simulink model "Obstacle_Detection"  (R2017b)
settings: configuration reference "Autosar_CodeGeneration" (kept outside this file)
settings Model: RequirementInfo={'linktype_rmi_url' 'http://md1hxhhc.ww004.siemens.net/polarion/' '@/project/ATRover/workitem?id=ATR-528' 'true' 'Polarion: ATR-528' '' } %GIDa_54e2749a_9850_4405_b077_57153701a047  DataDictionary=RoverDataDict.sldd  Creator=sam  LastModifiedBy=eh6qym
settings ConfigSetRef: DDName=RoverDataDict.sldd

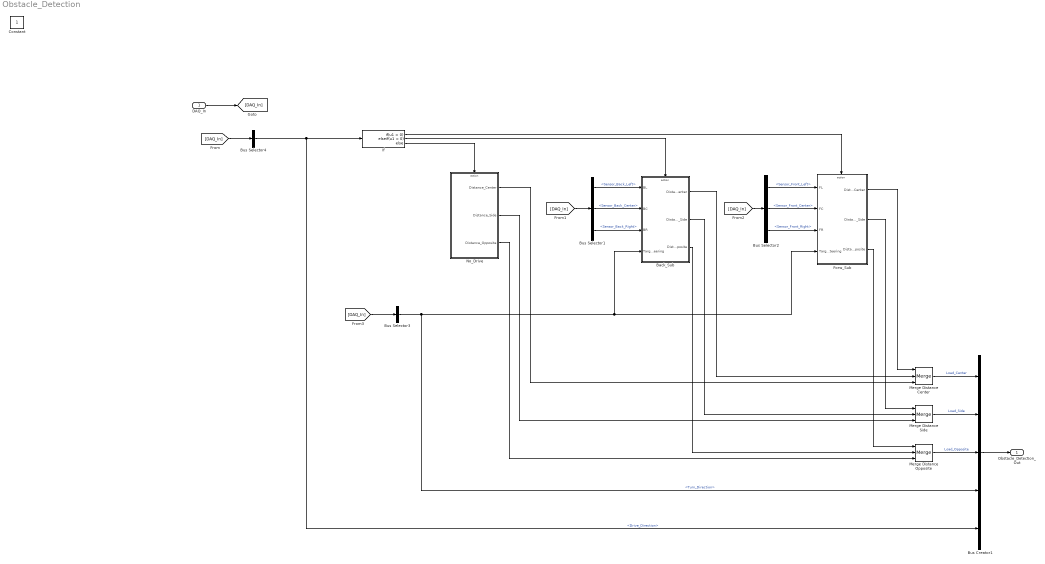
== system Obstacle_Detection ==
  DAQ_In : Inport  OutDataTypeStr=Bus: DAQ_In
  Back_Sub : Subsystem  TreatAsAtomicUnit=on
  Bus Creator1 : BusCreator  Inputs=5  OutDataTypeStr=Bus: Obstacle_Detection_Out  NonVirtualBus=on
      settings: InheritFromInputs=off
  Bus Selector1 : BusSelector  OutputSignals=Sensor_Back_Left,Sensor_Back_Center,Sensor_Back_Right
  Bus Selector2 : BusSelector  OutputSignals=Sensor_Front_Left,Sensor_Front_Center,Sensor_Front_Right
  Bus Selector3 : BusSelector  OutputSignals=Turn_Direction
  Bus Selector4 : BusSelector  OutputSignals=Drive_Direction
  Forw_Sub : Subsystem  TreatAsAtomicUnit=on
  If : If  ElseIfExpressions=u1 < 0
  Merge Distance Center : Merge  Inputs=3
  Merge Distance Opposite : Merge  Inputs=3
  Merge Distance Side : Merge  Inputs=3
  No_Drive : Subsystem  TreatAsAtomicUnit=on
  Obstacle_Detection_Out : Outport  OutDataTypeStr=Bus: Obstacle_Detection_Out
  Constant : Constant  IOType=siggen
  wires:
  Bus Creator1/1 -> Obstacle_Detection_Out/1
  Bus Selector1/1 -> Back_Sub/1(BL)  "<Sensor_Back_Left>"
  Bus Selector1/2 -> Back_Sub/2(BC)  "<Sensor_Back_Center>"
  Bus Selector1/3 -> Back_Sub/3(BR)  "<Sensor_Back_Right>"
  Bus Selector2/1 -> Forw_Sub/1(FL)  "<Sensor_Front_Left>"
  Bus Selector2/2 -> Forw_Sub/2(FC)  "<Sensor_Front_Center>"
  Bus Selector2/3 -> Forw_Sub/3(FR)  "<Sensor_Front_Right>"
  Bus Selector3/1 -> Bus Creator1/4, Forw_Sub/4(Target_Steering), Back_Sub/4(Target_Steering)  "<Turn_Direction>"
  Forw_Sub/2(Distance_Side) -> Merge Distance Side/1
  Back_Sub/2(Distance_Side) -> Merge Distance Side/2
  Merge Distance Side/1 -> Bus Creator1/2  "Load_Side"
  DAQ_In/1 -> [DAQ_In]
  [DAQ_In] -> Bus Selector4/1
  [DAQ_In] -> Bus Selector1/1
  [DAQ_In] -> Bus Selector2/1
  [DAQ_In] -> Bus Selector3/1
  Merge Distance Center/1 -> Bus Creator1/1  "Load_Center"
  Back_Sub/1(Distance_Center) -> Merge Distance Center/2
  Forw_Sub/1(Distance_Center) -> Merge Distance Center/1
  Bus Selector4/1 -> Bus Creator1/5, If/1  "<Drive_Direction>"
  If/1 -> Forw_Sub/Action
  If/2 -> Back_Sub/Action
  Merge Distance Opposite/1 -> Bus Creator1/3  "Load_Opposite"
  Forw_Sub/3(Distance_Opposite) -> Merge Distance Opposite/1
  Back_Sub/3(Distance_Opposite) -> Merge Distance Opposite/2
  If/3 -> No_Drive/Action
  No_Drive/1(Distance_Center) -> Merge Distance Center/3
  No_Drive/2(Distance_Side) -> Merge Distance Side/3
  No_Drive/3(Distance_Opposite) -> Merge Distance Opposite/3

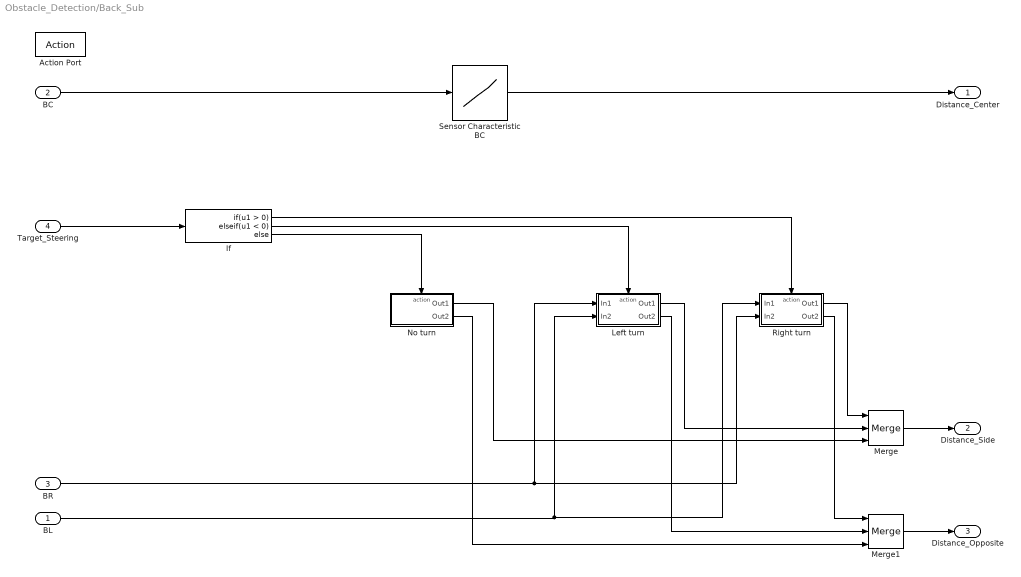
== system Obstacle_Detection/Back_Sub ==
  BL : Inport  OutDataTypeStr=double
  BC : Inport  Port=2  OutDataTypeStr=double
  BR : Inport  Port=3  OutDataTypeStr=double
  Target_Steering : Inport  Port=4  OutDataTypeStr=double
  Action Port : ActionPort  ActionType=elseif
  If : If  ElseIfExpressions=u1 < 0
  Left turn : Subsystem  TreatAsAtomicUnit=on
  Merge : Merge  Inputs=3
  Merge1 : Merge  Inputs=3
  No turn : Subsystem  TreatAsAtomicUnit=on
  Right turn : Subsystem  TreatAsAtomicUnit=on
  Sensor Characteristic BC : Lookup_n-D  NumberOfTableDimensions=1  BreakpointsForDimension1=[0.06 0.15 0.26 0.6 0.64]  Table=[0.80 0.40 0.20 0.07 0.06]  RemoveProtectionInput=on  InternalRulePriority=Speed  RndMeth=Simplest  InputSameDT=on
  Distance_Center : Outport  InitialOutput=[0.8]
  Distance_Side : Outport  Port=2  OutDataTypeStr=double  InitialOutput=[0.8]
  Distance_Opposite : Outport  Port=3  OutDataTypeStr=double  InitialOutput=[0.8]
  wires:
  BC/1 -> Sensor Characteristic BC/1
  Sensor Characteristic BC/1 -> Distance_Center/1
  Merge/1 -> Distance_Side/1
  BR/1 -> Right turn/2(In2), Left turn/1(In1)
  BL/1 -> Left turn/2(In2), Right turn/1(In1)
  Left turn/1(Out1) -> Merge/2
  Right turn/1(Out1) -> Merge/1
  If/1 -> Right turn/Action
  If/2 -> Left turn/Action
  Merge1/1 -> Distance_Opposite/1
  Left turn/2(Out2) -> Merge1/2
  Right turn/2(Out2) -> Merge1/1
  If/3 -> No turn/Action
  No turn/1(Out1) -> Merge/3
  No turn/2(Out2) -> Merge1/3
  Target_Steering/1 -> If/1

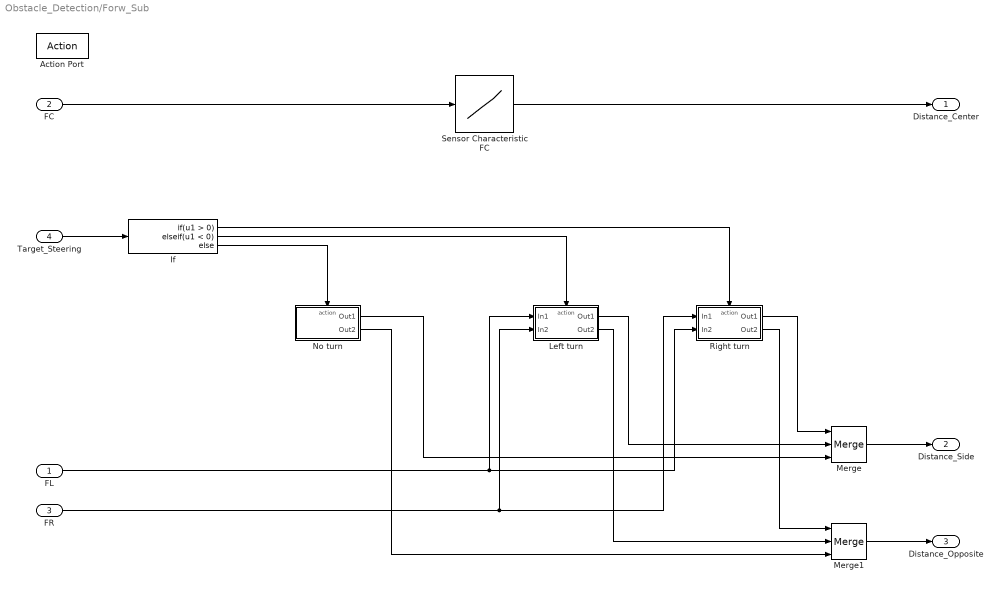
== system Obstacle_Detection/Forw_Sub ==
  FL : Inport  OutDataTypeStr=double
  FC : Inport  Port=2  OutDataTypeStr=double
  FR : Inport  Port=3  OutDataTypeStr=double
  Target_Steering : Inport  Port=4  OutDataTypeStr=double
  Action Port : ActionPort  ActionType=then
  If : If  ElseIfExpressions=u1 < 0
  Left turn : Subsystem  TreatAsAtomicUnit=on
  Merge : Merge  Inputs=3
  Merge1 : Merge  Inputs=3
  No turn : Subsystem  TreatAsAtomicUnit=on
  Right turn : Subsystem  TreatAsAtomicUnit=on
  Sensor Characteristic FC : Lookup_n-D  NumberOfTableDimensions=1  BreakpointsForDimension1=[0.06 0.15 0.26 0.6 0.64]  Table=[0.80 0.40 0.20 0.07 0.06]  RemoveProtectionInput=on  InternalRulePriority=Speed  RndMeth=Simplest  InputSameDT=on
  Distance_Center : Outport  InitialOutput=[0.8]
  Distance_Side : Outport  Port=2  OutDataTypeStr=double  InitialOutput=[0.8]
  Distance_Opposite : Outport  Port=3  OutDataTypeStr=double  InitialOutput=[0.8]
  wires:
  FC/1 -> Sensor Characteristic FC/1
  Sensor Characteristic FC/1 -> Distance_Center/1
  FR/1 -> Left turn/2(In2), Right turn/1(In1)
  FL/1 -> Right turn/2(In2), Left turn/1(In1)
  Right turn/1(Out1) -> Merge/1
  Left turn/1(Out1) -> Merge/2
  If/1 -> Right turn/Action
  If/2 -> Left turn/Action
  Merge1/1 -> Distance_Opposite/1
  Right turn/2(Out2) -> Merge1/1
  Left turn/2(Out2) -> Merge1/2
  No turn/1(Out1) -> Merge/3
  No turn/2(Out2) -> Merge1/3
  Target_Steering/1 -> If/1
  Merge/1 -> Distance_Side/1
  If/3 -> No turn/Action

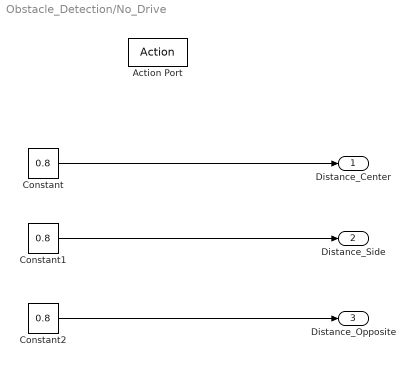
== system Obstacle_Detection/No_Drive ==
  Action Port : ActionPort  ActionType=else
  Constant : Constant  Value=0.8
  Constant1 : Constant  Value=0.8
  Constant2 : Constant  Value=0.8
  Distance_Center : Outport  InitialOutput=[0.8]
  Distance_Side : Outport  Port=2  OutDataTypeStr=double  InitialOutput=[0.8]
  Distance_Opposite : Outport  Port=3  OutDataTypeStr=double  InitialOutput=[0.8]
  wires:
  Constant/1 -> Distance_Center/1
  Constant1/1 -> Distance_Side/1
  Constant2/1 -> Distance_Opposite/1

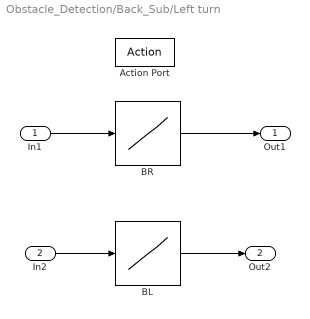
== system Obstacle_Detection/Back_Sub/Left turn ==
  In1 : Inport
  In2 : Inport  Port=2
  Action Port : ActionPort  ActionType=elseif
  BL : Lookup_n-D  NumberOfTableDimensions=1  BreakpointsForDimension1=[0.06 0.15 0.26 0.6 0.64]  Table=[0.80 0.40 0.20 0.07 0.06]  RemoveProtectionInput=on  InternalRulePriority=Speed  RndMeth=Simplest  InputSameDT=on
  BR : Lookup_n-D  NumberOfTableDimensions=1  BreakpointsForDimension1=[0.06 0.15 0.26 0.6 0.64]  Table=[0.80 0.40 0.20 0.07 0.06]  RemoveProtectionInput=on  InternalRulePriority=Speed  RndMeth=Simplest  InputSameDT=on
  Out1 : Outport  InitialOutput=[0.8]
  Out2 : Outport  Port=2  InitialOutput=[0.8]
  wires:
  In1/1 -> BR/1
  BR/1 -> Out1/1
  In2/1 -> BL/1
  BL/1 -> Out2/1

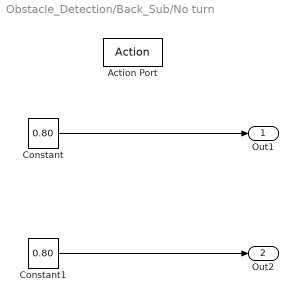
== system Obstacle_Detection/Back_Sub/No turn ==
  Action Port : ActionPort  ActionType=else
  Constant : Constant  Value=0.80
  Constant1 : Constant  Value=0.80
  Out1 : Outport  InitialOutput=[0.8]
  Out2 : Outport  Port=2  InitialOutput=[0.8]
  wires:
  Constant/1 -> Out1/1
  Constant1/1 -> Out2/1

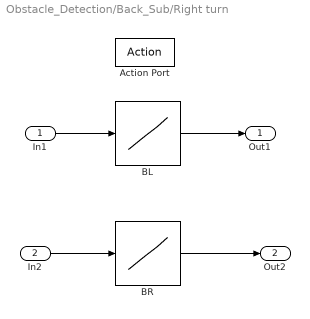
== system Obstacle_Detection/Back_Sub/Right turn ==
  In1 : Inport
  In2 : Inport  Port=2
  Action Port : ActionPort  ActionType=then
  BL : Lookup_n-D  NumberOfTableDimensions=1  BreakpointsForDimension1=[0.06 0.15 0.26 0.6 0.64]  Table=[0.80 0.40 0.20 0.07 0.06]  RemoveProtectionInput=on  InternalRulePriority=Speed  RndMeth=Simplest  InputSameDT=on
  BR : Lookup_n-D  NumberOfTableDimensions=1  BreakpointsForDimension1=[0.06 0.15 0.26 0.6 0.64]  Table=[0.80 0.40 0.20 0.07 0.06]  RemoveProtectionInput=on  InternalRulePriority=Speed  RndMeth=Simplest  InputSameDT=on
  Out1 : Outport  InitialOutput=[0.8]
  Out2 : Outport  Port=2  InitialOutput=[0.8]
  wires:
  In1/1 -> BL/1
  BL/1 -> Out1/1
  In2/1 -> BR/1
  BR/1 -> Out2/1

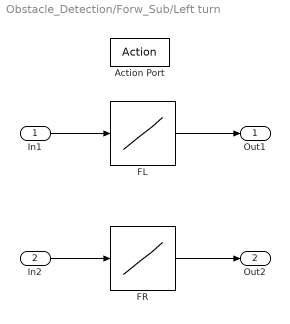
== system Obstacle_Detection/Forw_Sub/Left turn ==
  In1 : Inport
  In2 : Inport  Port=2
  Action Port : ActionPort  ActionType=elseif
  FL : Lookup_n-D  NumberOfTableDimensions=1  BreakpointsForDimension1=[0.06 0.15 0.26 0.6 0.64]  Table=[0.80 0.40 0.20 0.07 0.06]  RemoveProtectionInput=on  InternalRulePriority=Speed  RndMeth=Simplest  InputSameDT=on
  FR : Lookup_n-D  NumberOfTableDimensions=1  BreakpointsForDimension1=[0.06 0.15 0.26 0.6 0.64]  Table=[0.80 0.40 0.20 0.07 0.06]  RemoveProtectionInput=on  InternalRulePriority=Speed  RndMeth=Simplest  InputSameDT=on
  Out1 : Outport  InitialOutput=[0.8]
  Out2 : Outport  Port=2  InitialOutput=[0.8]
  wires:
  In1/1 -> FL/1
  FL/1 -> Out1/1
  In2/1 -> FR/1
  FR/1 -> Out2/1

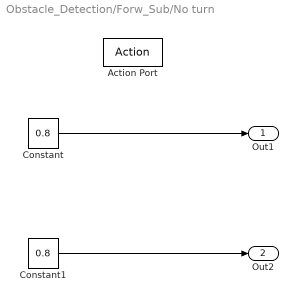
== system Obstacle_Detection/Forw_Sub/No turn ==
  Action Port : ActionPort  ActionType=else
  Constant : Constant  Value=0.8
  Constant1 : Constant  Value=0.8
  Out1 : Outport  InitialOutput=[0.8]
  Out2 : Outport  Port=2  InitialOutput=[0.8]
  wires:
  Constant/1 -> Out1/1
  Constant1/1 -> Out2/1

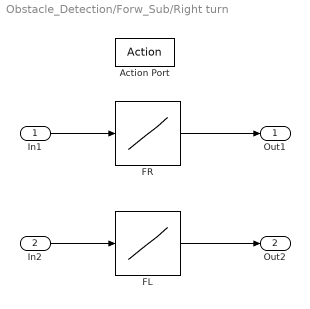
== system Obstacle_Detection/Forw_Sub/Right turn ==
  In1 : Inport
  In2 : Inport  Port=2
  Action Port : ActionPort  ActionType=then
  FL : Lookup_n-D  NumberOfTableDimensions=1  BreakpointsForDimension1=[0.06 0.15 0.26 0.6 0.64]  Table=[0.80 0.40 0.20 0.07 0.06]  RemoveProtectionInput=on  InternalRulePriority=Speed  RndMeth=Simplest  InputSameDT=on
  FR : Lookup_n-D  NumberOfTableDimensions=1  BreakpointsForDimension1=[0.06 0.15 0.26 0.6 0.64]  Table=[0.80 0.40 0.20 0.07 0.06]  RemoveProtectionInput=on  InternalRulePriority=Speed  RndMeth=Simplest  InputSameDT=on
  Out1 : Outport  InitialOutput=[0.8]
  Out2 : Outport  Port=2  InitialOutput=[0.8]
  wires:
  In1/1 -> FR/1
  FR/1 -> Out1/1
  In2/1 -> FL/1
  FL/1 -> Out2/1
